simulink model "simulation2023a"  (R2023b)
settings: Solver=FixedStepAuto  StartTime=0.0  StopTime=10  FixedStep=T_vz  RelTol=1e-3
values from neighbouring files (symbols this model uses):
  B_e = 0.05    [GA.m]    (also in exam.m = 0.001; grafs.m = gears(i); pi_GA.m; test.m = 0.001)
  B_m = 0.000080292    (= 8.0292e-05)    [GA.m]    (also in exam.m; pi_GA.m; test.m)
  B_z = 0.00020000    (= 0.0002)    [GA.m]    (also in exam.m; pi_GA.m; test.m)
  i = 5    [exam.m]
  J_m = 0.00009    (= 9e-05)    [GA.m]    (also in exam.m; pi_GA.m; test.m)
  J_z = 0.00024943    [GA.m]    (also in exam.m; pi_GA.m; test.m)
  K_e = 0.5    [GA.m]    (also in exam.m = 0.01; grafs.m = gears(i); pi_GA.m; test.m = 0.01)
  M_z0m = 0.0052    [GA.m]    (also in exam.m; pi_GA.m; test.m)
  N_el = 10000    [GA.m]    (also in exam.m; pi_GA.m; test.m)
  T_n = 0.001    [GA.m]    (also in exam.m; pi_GA.m; test.m)
  T_vz = 0.001    [GA.m]    (also in exam.m; pi_GA.m; test.m)
undefined symbols (not defined in the file or in its folder): I, P
libraries: slpidlib x1, SignalEditorBlockLib x1
settings Model: Creator=laptop  LastModifiedBy=maros-pc
settings SolverCC: ConsecutiveZCsStepRelTol=10000*128*eps  EnableFixedStepZeroCrossing=on  MaxZcPerStep=10

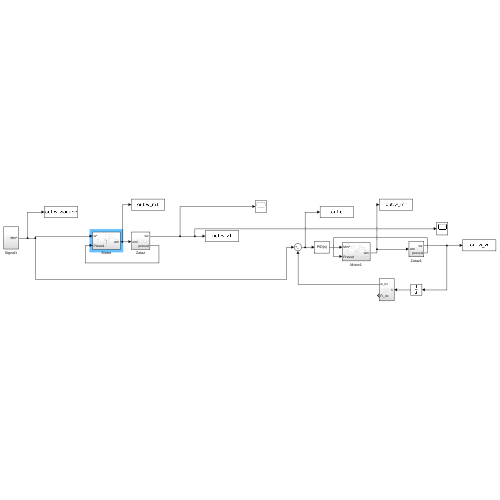
[thumbnail: Simulink's stored preview of the top-level diagram]
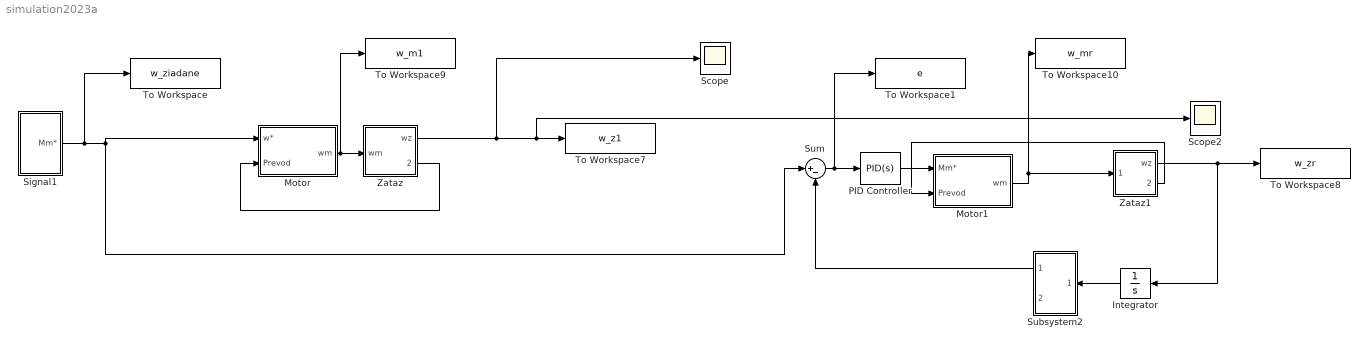
== system simulation2023a ==
  Integrator : Integrator
  Motor : Subsystem
  Motor1 : Subsystem
  PID Controller : slpidlib/PID Controller  Controller=PID  Form=Parallel  TimeDomain=Continuous-time  UseExternalTs=off  SampleTime=-1  IntegratorMethod=Forward Euler  FilterMethod=Forward Euler  ControllerParametersSource=internal  P=P  I=I  UseKiTs=off  D=0  N=100  UseFilter=on  TunerSelectOption=Transfer Function Based (PID Tuner App)  InitialConditionSource=internal  InitialConditionForIntegrator=0  InitialConditionForFilter=0  DifferentiatorICPrevScaledInput=0  ExternalReset=none  TrackingMode=off  Kt=1  LimitOutput=off  SatLimitsSource=internal  UpperSaturationLimit=inf  LowerSaturationLimit=-inf  LinearizeAsGain=on  AntiWindupMode=none  Kb=1  LimitIntegrator=off  UpperIntegratorSaturationLimit=inf  LowerIntegratorSaturationLimit=-inf  POutMin=[]  POutMax=[]  IOutMin=[]  IOutMax=[]  DOutMin=[]  DOutMax=[]  NOutMin=[]  NOutMax=[]  SumOutMin=[]  SumOutMax=[]  SaturationOutMin=[]  SaturationOutMax=[]  PParamMin=[]  PParamMax=[]  IParamMin=[]  IParamMax=[]  DParamMin=[]  DParamMax=[]  NParamMin=[]  NParamMax=[]  KbParamMin=[]  KbParamMax=[]  KtParamMin=[]  KtParamMax=[]  KbOutMin=[]  KbOutMax=[]  KtOutMin=[]  KtOutMax=[]  IntegratorOutMin=[]  IntegratorOutMax=[]  FilterOutMin=[]  FilterOutMax=[]  SumI1OutMin=[]  SumI1OutMax=[]  SumI2OutMin=[]  SumI2OutMax=[]  SumI3OutMin=[]  SumI3OutMax=[]  SumI4OutMin=[]  SumI4OutMax=[]  SumDOutMin=[]  SumDOutMax=[]  DifferentiatorOutMin=[]  DifferentiatorOutMax=[]  FilterDiffOutCoefMin=[]  FilterDiffOutCoefMax=[]  ReciprocalOutMin=[]  ReciprocalOutMax=[]  SumDenOutMin=[]  SumDenOutMax=[]  SumNumOutMin=[]  SumNumOutMax=[]  DivideOutMin=[]  DivideOutMax=[]  UdiffTsProdOutMin=[]  UdiffTsProdOutMax=[]  NTsProdOutMin=[]  NTsProdOutMax=[]  UintegralTsProdOutMin=[]  UintegralTsProdOutMax=[]  UngainTsProdOutMin=[]  UngainTsProdOutMax=[]  ClampingZeroOutDataTypeStr=Inherit: Inherit via back propagation  ClampingZeroOutMin=[]  ClampingZeroOutMax=[]  FilterDenConstantOutDataTypeStr=Inherit: Inherit via back propagation  FilterDenConstantOutMin=[]  FilterDenConstantOutMax=[]  PCopyOutDataTypeStr=Inherit: Inherit via back propagation  PCopyOutMin=[]  PCopyOutMax=[]  NCopyOutDataTypeStr=Inherit: Inherit via back propagation  NCopyOutMin=[]  NCopyOutMax=[]  IntegratorContinuousStateAttributes=''  IntegratorStateMustResolveToSignalObject=off  IntegratorRTWStateStorageClass=Auto  FilterContinuousStateAttributes=''  FilterStateMustResolveToSignalObject=off  FilterRTWStateStorageClass=Auto  ParallelPVariant=InternalParameters  IdealPVariant=Disabled  IVariant=InternalParameters  DVariant=InternalParameters  IntegratorVariant=Continuous  SatVariant=Disabled  AWVariant=Passthrough  PCopyVariant=Disabled  TRVariant=Disabled  FdbkBlocksVariant=Forward  IdealPFdbkVariant=Disabled  SatFdbkVariant=Disabled  DerivativeFilterVariant=ContFilter  NVariant=InternalParameters  NCopyVariant=Disabled  FilterICVariant=InternalICsFilter  IntegratorICVariant=InternalICs  ExternalResetVariant=Disabled  TRSumVariant=Passthrough  SumFdbkVariant=Disabled  SumVariant=Sum_PID  TsampFilterVariant=InternalTs  TsampNgainVariant=Passthrough  TsampIntegralVariant=Disabled_SignalSpec  ExternalSaturationOutDataTypeStr=Inherit: Same as second input
  Scope : Scope
  Scope2 : Scope
  Signal1 : Subsystem
  Subsystem2 : Subsystem
  Sum : Sum  Inputs=|+-
  To Workspace : ToWorkspace  VariableName=w_ziadane  SaveFormat=Timeseries  SampleTime=-1
  To Workspace1 : ToWorkspace  VariableName=e  SaveFormat=Timeseries  SampleTime=-1
  To Workspace10 : ToWorkspace  VariableName=w_mr  SaveFormat=Timeseries  SampleTime=-1
  To Workspace7 : ToWorkspace  VariableName=w_z1  SaveFormat=Timeseries  SampleTime=-1
  To Workspace8 : ToWorkspace  VariableName=w_zr  SaveFormat=Timeseries  SampleTime=-1
  To Workspace9 : ToWorkspace  VariableName=w_m1  SaveFormat=Timeseries  SampleTime=-1
  Zataz : Subsystem
  Zataz1 : Subsystem
  wires:
  Signal1/1(Mm*) -> To Workspace/1, Motor/1(w*), Sum/1
  Motor/1(wm) -> To Workspace9/1, Zataz/1(wm)
  Zataz/1(wz) -> Scope2/1, To Workspace7/1, Scope/1
  Zataz/2(prevod) -> Motor/2(Prevod)
  Zataz1/2(prevod) -> Motor1/2(Prevod)
  Zataz1/1(wz) -> Integrator/1, To Workspace8/1
  Motor1/1(wm) -> To Workspace10/1, Zataz1/1(wm)
  Integrator/1 -> Subsystem2/1(In1)
  PID Controller/1 -> Motor1/1(Mm*)
  Sum/1 -> To Workspace1/1, PID Controller/1
  Subsystem2/1(w_irc) -> Sum/2

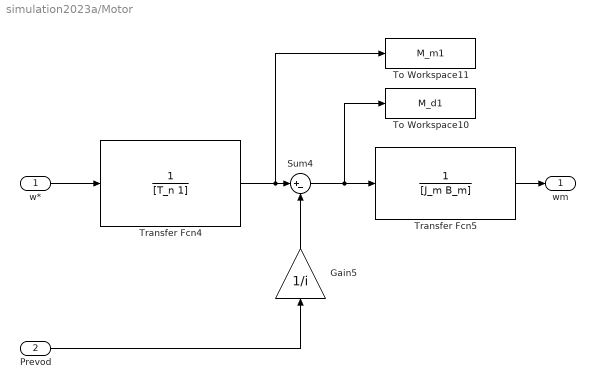
== system simulation2023a/Motor ==
  w* : Inport
  Prevod : Inport  Port=2
  Gain5 : Gain  Gain=1/i
  Sum4 : Sum  Inputs=|+-
  To Workspace10 : ToWorkspace  VariableName=M_d1  SaveFormat=Timeseries  SampleTime=-1
  To Workspace11 : ToWorkspace  VariableName=M_m1  SaveFormat=Timeseries  SampleTime=-1
  Transfer Fcn4 : TransferFcn  Denominator=[T_n 1]
  Transfer Fcn5 : TransferFcn  Denominator=[J_m B_m]
  wm : Outport
  wires:
  Gain5/1 -> Sum4/2
  Sum4/1 -> To Workspace10/1, Transfer Fcn5/1
  Transfer Fcn4/1 -> To Workspace11/1, Sum4/1
  w*/1 -> Transfer Fcn4/1
  Prevod/1 -> Gain5/1
  Transfer Fcn5/1 -> wm/1

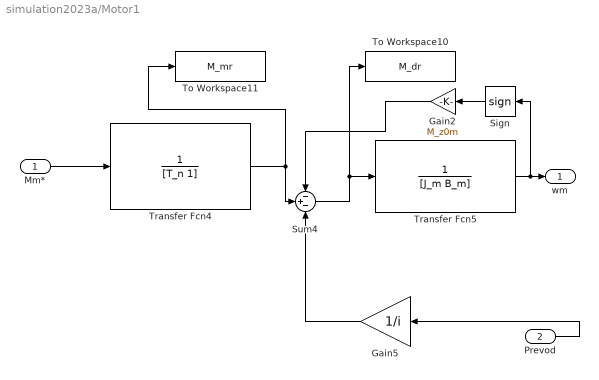
== system simulation2023a/Motor1 ==
  Mm* : Inport
  Prevod : Inport  Port=2
  Gain2 : Gain  Gain=M_z0m
  Gain5 : Gain  Gain=1/i
  Sign : Signum
  Sum4 : Sum  Inputs=-+-
  To Workspace10 : ToWorkspace  VariableName=M_dr  SaveFormat=Timeseries  SampleTime=-1
  To Workspace11 : ToWorkspace  VariableName=M_mr  SaveFormat=Timeseries  SampleTime=-1
  Transfer Fcn4 : TransferFcn  Denominator=[T_n 1]
  Transfer Fcn5 : TransferFcn  Denominator=[J_m B_m]
  wm : Outport
  wires:
  Gain5/1 -> Sum4/3
  Sum4/1 -> To Workspace10/1, Transfer Fcn5/1
  Transfer Fcn4/1 -> Sum4/2, To Workspace11/1
  Mm*/1 -> Transfer Fcn4/1
  Prevod/1 -> Gain5/1
  Gain2/1 -> Sum4/1
  Sign/1 -> Gain2/1
  Transfer Fcn5/1 -> Sign/1, wm/1

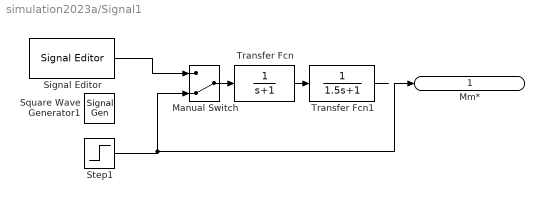
== system simulation2023a/Signal1 ==
  Manual Switch : ManualSwitch  CurrentSetting=0
  Signal Editor : SignalEditorBlockLib/Signal Editor  FileName=signal.mat  ActiveScenario=Scenario  ActiveSignal=Signal 1  IsBus=off  OutputBusObjectStr=Bus: BusObject  SampleTime=0  Interpolate=off  ZeroCross=off  OutputAfterFinalValue=Setting to zero  Unit=inherit  PreserveSignalName=on  ApplySigPropsToAllScenarios=on  ApplySigPropsToAllSignals=off
  Square Wave Generator1 : SignalGenerator  WaveForm=sawtooth  Amplitude=2  Frequency=10
  Step1 : Step  After=2*pi  SampleTime=0
  Transfer Fcn : TransferFcn  Denominator=[1 1]
  Transfer Fcn1 : TransferFcn  Denominator=[1.5 1]
  Mm* : Outport
  wires:
  Manual Switch/1 -> Transfer Fcn/1
  Step1/1 -> Mm*/1, Manual Switch/2
  Signal Editor/1 -> Manual Switch/1
  Transfer Fcn/1 -> Transfer Fcn1/1
  Transfer Fcn1/1 -> ?

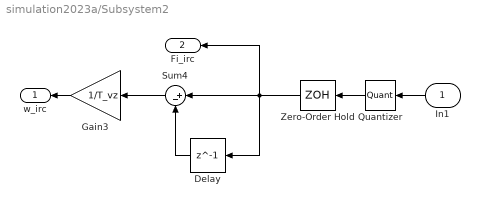
== system simulation2023a/Subsystem2 ==
  In1 : Inport
  Delay : Delay  DelayLength=1
  Gain3 : Gain  Gain=1/T_vz
  Quantizer : Quantizer  QuantizationInterval=2*pi/N_el
  Sum4 : Sum  Inputs=|+-
  Zero-Order Hold : ZeroOrderHold  SampleTime=T_vz
  w_irc : Outport
  Fi_irc : Outport  Port=2
  wires:
  Sum4/1 -> Gain3/1
  Delay/1 -> Sum4/2
  Zero-Order Hold/1 -> Delay/1, Sum4/1, Fi_irc/1
  In1/1 -> Quantizer/1
  Quantizer/1 -> Zero-Order Hold/1
  Gain3/1 -> w_irc/1

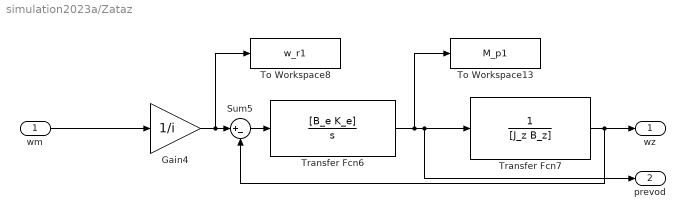
== system simulation2023a/Zataz ==
  wm : Inport
  Gain4 : Gain  Gain=1/i
  Sum5 : Sum  Inputs=|+-
  To Workspace13 : ToWorkspace  VariableName=M_p1  SaveFormat=Timeseries  SampleTime=-1
  To Workspace8 : ToWorkspace  VariableName=w_r1  SaveFormat=Timeseries  SampleTime=-1
  Transfer Fcn6 : TransferFcn  Numerator=[B_e K_e]  Denominator=[1 0]
  Transfer Fcn7 : TransferFcn  Denominator=[J_z B_z]
  wz : Outport
  prevod : Outport  Port=2
  wires:
  wm/1 -> Gain4/1
  Sum5/1 -> Transfer Fcn6/1
  Transfer Fcn6/1 -> To Workspace13/1, prevod/1, Transfer Fcn7/1
  Gain4/1 -> To Workspace8/1, Sum5/1
  Transfer Fcn7/1 -> wz/1, Sum5/2

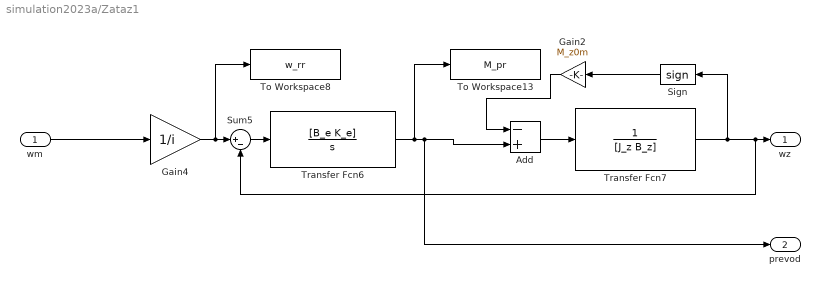
== system simulation2023a/Zataz1 ==
  wm : Inport
  Add : Sum  Inputs=-+
  Gain2 : Gain  Gain=M_z0m
  Gain4 : Gain  Gain=1/i
  Sign : Signum
  Sum5 : Sum  Inputs=|+-
  To Workspace13 : ToWorkspace  VariableName=M_pr  SaveFormat=Timeseries  SampleTime=-1
  To Workspace8 : ToWorkspace  VariableName=w_rr  SaveFormat=Timeseries  SampleTime=-1
  Transfer Fcn6 : TransferFcn  Numerator=[B_e K_e]  Denominator=[1 0]
  Transfer Fcn7 : TransferFcn  Denominator=[J_z B_z]
  wz : Outport
  prevod : Outport  Port=2
  wires:
  wm/1 -> Gain4/1
  Sum5/1 -> Transfer Fcn6/1
  Transfer Fcn6/1 -> To Workspace13/1, Add/2, prevod/1
  Gain4/1 -> To Workspace8/1, Sum5/1
  Transfer Fcn7/1 -> Sign/1, Sum5/2, wz/1
  Gain2/1 -> Add/1
  Sign/1 -> Gain2/1
  Add/1 -> Transfer Fcn7/1
